simulink model "Basics"  (R2019a)
settings: Solver=ode1  StartTime=0.0  StopTime=2.5  FixedStep=Ts_Power  RelTol=1e-3
PostLoadFcn:
  | %% Init for wind PnO models - global system parameters
  | OVERRIDE_SSN_MEMORY_LIMIT=1;
  | Ts=50e-6;
  | % Ts=50e-10;
  | Ts_Power=Ts;
  | Ts_Control=2*Ts;
  | freq = 50;
  | Fnom=freq;
  | Vac=400e3;
InitFcn:
  | %% Init for wind PnO models - global system parameters
  | OVERRIDE_SSN_MEMORY_LIMIT=1;
  | Ts=50e-6;
  | % Ts=50e-10;
  | Ts_Power=Ts;
  | Ts_Control=2*Ts;
  | freq = 50;
  | Fnom=freq;
  | Vac=225e3;
values from neighbouring files (symbols this model uses):
  ohl_posCap = 11.33e-009/2    (= 5.665e-09)    [variable.m]
  ohl_posInd = 1.05e-3/2    (= 0.000525)    [variable.m]
  ohl_posR = 0.1153/2    (= 0.05765)    [variable.m]
  ohl_zeroCap = 5.01e-009/2    (= 2.505e-09)    [variable.m]
  ohl_zeroInd = 3.32e-3/2    (= 0.00166)    [variable.m]
  ohl_zeroR = 0.4138/2    (= 0.2069)    [variable.m]
  sub_posCap = 0.16e-006    (= 1.6e-07)    [variable.m]
  sub_posInd = 0.001400563    [variable.m]
  sub_posR = 0.036    [variable.m]
  sub_zeroCap = 0.053333e-006    (= 5.3333e-08)    [variable.m]
  sub_zeroInd = 0.00420169    [variable.m]
  sub_zeroR = 0.108    [variable.m]
  transfo_L1 = 0.05999374    [variable.m]
  transfo_L2 = 0.05999374    [variable.m]
  transfo_R1 = 0.000866667    [variable.m]
  transfo_R2 = 0.00086667    [variable.m]
undefined symbols (not defined in the file or in its folder): D1, D11, Delta, den, DiscIntNeverNeededParam, dx, find_system, gcbh, num, out_Buses, out_WindFarms, sps_rtmsupport
libraries: powerlib x173, simulink x80, powerlib_meascontrol x80, elements x52, eeSinusoidalMeasurement x46, simulink_extras x40, spsVIMeasurementModel x36, eePowerMeasurement x15
(part 21 of 22)

== system Basics/SM_WT1/Wind Type IV Detailed v2.1 - 3/Control/Measurement and Transformation/Discrete 3-phase PLL-Driven Positive-Sequence Active & Reactive Power/Discrete 3-phase PLL-Driven Positive-Sequence Fundamental Value/Discrete Variable Frequency Mean value1 ==
  note: Pierre Giroux, Gilbert Sybille, Richard Gagnon
      | Power System Simulation Laboratory
      | IREQ, Hydro-Quebc
  note: Variable frequency - Discrete Mean Value
  Freq : Inport  PortDimensions=1
  In : Inport  Port=2  PortDimensions=1
  Correction subsystem : Subsystem
  Discrete Variable Transport Delay : Subsystem  mask(Discrete variable transport delay){MaxDelay=MaxDelay, InitialValue=0, Ts=Ts}
      mask prompts: MaxDelay "Maximum delay (s):"; InitialValue "Initial input:"; Ts "Sample time:"
      mask help:
      | Apply a delay to the first input (In) signal.
      | The second input (D) specifies the delay time.
  Gain : Gain  Gain=Ts  SaturateOnIntegerOverflow=on  OutDataTypeStr=Inherit: Same as input  ParamDataTypeStr=Inherit: Same as input
  Integ4 : DiscreteIntegrator  IntegratorMethod=Integration: Trapezoidal  SampleTime=Ts  ICPrevOutput=DiscIntNeverNeededParam  ICPrevScaledInput=DiscIntNeverNeededParam
  Number of samples per cycle : Fcn  Expr=1/u[1]/Ts
  Product : Product  SaturateOnIntegerOverflow=on  InputSameDT=on  OutDataTypeStr=Inherit: Same as first input
  Rounding Function : Rounding  Operator=ceil
  Step : Step  Time=1/Finit  SampleTime=Ts
  Sum5 : Sum  SaturateOnIntegerOverflow=on  InputSameDT=on  OutDataTypeStr=Inherit: Same as first input
  Sum7 : Sum  Inputs=-+  SaturateOnIntegerOverflow=on  InputSameDT=on  OutDataTypeStr=Inherit: Same as first input
  Switch : Switch  Threshold=0.5  InputSameDT=on
  To avoid division by zero : Saturate  UpperLimit=1e6  LowerLimit=1e-6
  Unit Delay : UnitDelay  InitialCondition=Vinit  SampleTime=Ts  HasFrameUpgradeWarning=on
  Mean : Outport  VectorParamsAs1DForOutWhenUnconnected=on
  wires:
  In/1 -> Integ4/1, Correction subsystem/3(In)  "In"
  Product/1 -> Sum5/1  "Mean value"
  Discrete Variable Transport Delay/1(Out) -> Sum7/1
  Sum7/1 -> Product/1
  Integ4/1 -> Discrete Variable Transport Delay/1(In), Sum7/2
  Freq/1 -> Product/2, To avoid division by zero/1  "Freq"
  Gain/1 -> Discrete Variable Transport Delay/2(D)  "Delay"
  Rounding Function/1 -> Gain/1, Correction subsystem/2(F)
  Number of samples per cycle/1 -> Rounding Function/1, Correction subsystem/1(N)
  Sum5/1 -> Switch/1
  Unit Delay/1 -> Switch/3
  Switch/1 -> Mean/1, Unit Delay/1
  To avoid division by zero/1 -> Number of samples per cycle/1  "Freq"
  Correction subsystem/1(Out) -> Sum5/2
  Step/1 -> Switch/2

== system Basics/SM_WT1/Wind Type IV Detailed v2.1 - 3/Control/Measurement and Transformation/Discrete 3-phase PLL-Driven Positive-Sequence Active & Reactive Power/Discrete 3-phase PLL-Driven Positive-Sequence Fundamental Value/Discrete Variable Frequency Mean value2 ==
  note: Variable frequency - Discrete Mean Value
  note: Pierre Giroux, Gilbert Sybille, Richard Gagnon
      | Power System Simulation Laboratory
      | IREQ, Hydro-Quebc
  Freq : Inport  PortDimensions=1
  In : Inport  Port=2  PortDimensions=1
  Correction subsystem : Subsystem
  Discrete Variable Transport Delay : Subsystem  mask(Discrete variable transport delay){MaxDelay=MaxDelay, InitialValue=0, Ts=Ts}
      mask prompts: MaxDelay "Maximum delay (s):"; InitialValue "Initial input:"; Ts "Sample time:"
      mask help:
      | Apply a delay to the first input (In) signal.
      | The second input (D) specifies the delay time.
  Gain : Gain  Gain=Ts  SaturateOnIntegerOverflow=on  OutDataTypeStr=Inherit: Same as input  ParamDataTypeStr=Inherit: Same as input
  Integ4 : DiscreteIntegrator  IntegratorMethod=Integration: Trapezoidal  SampleTime=Ts  ICPrevOutput=DiscIntNeverNeededParam  ICPrevScaledInput=DiscIntNeverNeededParam
  Number of samples per cycle : Fcn  Expr=1/u[1]/Ts
  Product : Product  SaturateOnIntegerOverflow=on  InputSameDT=on  OutDataTypeStr=Inherit: Same as first input
  Rounding Function : Rounding  Operator=ceil
  Step : Step  Time=1/Finit  SampleTime=Ts
  Sum5 : Sum  SaturateOnIntegerOverflow=on  InputSameDT=on  OutDataTypeStr=Inherit: Same as first input
  Sum7 : Sum  Inputs=-+  SaturateOnIntegerOverflow=on  InputSameDT=on  OutDataTypeStr=Inherit: Same as first input
  Switch : Switch  Threshold=0.5  InputSameDT=on
  To avoid division by zero : Saturate  UpperLimit=1e6  LowerLimit=1e-6
  Unit Delay : UnitDelay  InitialCondition=Vinit  SampleTime=Ts  HasFrameUpgradeWarning=on
  Mean : Outport  VectorParamsAs1DForOutWhenUnconnected=on
  wires:
  Step/1 -> Switch/2
  Correction subsystem/1(Out) -> Sum5/2
  To avoid division by zero/1 -> Number of samples per cycle/1  "Freq"
  Switch/1 -> Unit Delay/1, Mean/1
  Unit Delay/1 -> Switch/3
  Sum5/1 -> Switch/1
  Number of samples per cycle/1 -> Correction subsystem/1(N), Rounding Function/1
  Rounding Function/1 -> Correction subsystem/2(F), Gain/1
  Gain/1 -> Discrete Variable Transport Delay/2(D)  "Delay"
  Freq/1 -> To avoid division by zero/1, Product/2  "Freq"
  Integ4/1 -> Sum7/2, Discrete Variable Transport Delay/1(In)
  Sum7/1 -> Product/1
  Discrete Variable Transport Delay/1(Out) -> Sum7/1
  Product/1 -> Sum5/1  "Mean value"
  In/1 -> Correction subsystem/3(In), Integ4/1  "In"

== system Basics/SM_WT1/Wind Type IV Detailed v2.1 - 3/Control/Measurement and Transformation/Discrete 3-phase PLL-Driven Positive-Sequence Active & Reactive Power/Discrete 3-phase PLL-Driven Positive-Sequence Fundamental Value2/Discrete Variable Frequency Mean value1 ==
  note: Variable frequency - Discrete Mean Value
  note: Pierre Giroux, Gilbert Sybille, Richard Gagnon
      | Power System Simulation Laboratory
      | IREQ, Hydro-Quebc
  Freq : Inport  PortDimensions=1
  In : Inport  Port=2  PortDimensions=1
  Correction subsystem : Subsystem
  Discrete Variable Transport Delay : Subsystem  mask(Discrete variable transport delay){MaxDelay=MaxDelay, InitialValue=0, Ts=Ts}
      mask prompts: MaxDelay "Maximum delay (s):"; InitialValue "Initial input:"; Ts "Sample time:"
      mask help:
      | Apply a delay to the first input (In) signal.
      | The second input (D) specifies the delay time.
  Gain : Gain  Gain=Ts  SaturateOnIntegerOverflow=on  OutDataTypeStr=Inherit: Same as input  ParamDataTypeStr=Inherit: Same as input
  Integ4 : DiscreteIntegrator  IntegratorMethod=Integration: Trapezoidal  SampleTime=Ts  ICPrevOutput=DiscIntNeverNeededParam  ICPrevScaledInput=DiscIntNeverNeededParam
  Number of samples per cycle : Fcn  Expr=1/u[1]/Ts
  Product : Product  SaturateOnIntegerOverflow=on  InputSameDT=on  OutDataTypeStr=Inherit: Same as first input
  Rounding Function : Rounding  Operator=ceil
  Step : Step  Time=1/Finit  SampleTime=Ts
  Sum5 : Sum  SaturateOnIntegerOverflow=on  InputSameDT=on  OutDataTypeStr=Inherit: Same as first input
  Sum7 : Sum  Inputs=-+  SaturateOnIntegerOverflow=on  InputSameDT=on  OutDataTypeStr=Inherit: Same as first input
  Switch : Switch  Threshold=0.5  InputSameDT=on
  To avoid division by zero : Saturate  UpperLimit=1e6  LowerLimit=1e-6
  Unit Delay : UnitDelay  InitialCondition=Vinit  SampleTime=Ts  HasFrameUpgradeWarning=on
  Mean : Outport  VectorParamsAs1DForOutWhenUnconnected=on
  wires:
  Step/1 -> Switch/2
  Correction subsystem/1(Out) -> Sum5/2
  To avoid division by zero/1 -> Number of samples per cycle/1  "Freq"
  Switch/1 -> Unit Delay/1, Mean/1
  Unit Delay/1 -> Switch/3
  Sum5/1 -> Switch/1
  Number of samples per cycle/1 -> Correction subsystem/1(N), Rounding Function/1
  Rounding Function/1 -> Correction subsystem/2(F), Gain/1
  Gain/1 -> Discrete Variable Transport Delay/2(D)  "Delay"
  Freq/1 -> To avoid division by zero/1, Product/2  "Freq"
  Integ4/1 -> Sum7/2, Discrete Variable Transport Delay/1(In)
  Sum7/1 -> Product/1
  Discrete Variable Transport Delay/1(Out) -> Sum7/1
  Product/1 -> Sum5/1  "Mean value"
  In/1 -> Correction subsystem/3(In), Integ4/1  "In"

== system Basics/SM_WT1/Wind Type IV Detailed v2.1 - 3/Control/Measurement and Transformation/Discrete 3-phase PLL-Driven Positive-Sequence Active & Reactive Power/Discrete 3-phase PLL-Driven Positive-Sequence Fundamental Value2/Discrete Variable Frequency Mean value2 ==
  note: Pierre Giroux, Gilbert Sybille, Richard Gagnon
      | Power System Simulation Laboratory
      | IREQ, Hydro-Quebc
  note: Variable frequency - Discrete Mean Value
  Freq : Inport  PortDimensions=1
  In : Inport  Port=2  PortDimensions=1
  Correction subsystem : Subsystem
  Discrete Variable Transport Delay : Subsystem  mask(Discrete variable transport delay){MaxDelay=MaxDelay, InitialValue=0, Ts=Ts}
      mask prompts: MaxDelay "Maximum delay (s):"; InitialValue "Initial input:"; Ts "Sample time:"
      mask help:
      | Apply a delay to the first input (In) signal.
      | The second input (D) specifies the delay time.
  Gain : Gain  Gain=Ts  SaturateOnIntegerOverflow=on  OutDataTypeStr=Inherit: Same as input  ParamDataTypeStr=Inherit: Same as input
  Integ4 : DiscreteIntegrator  IntegratorMethod=Integration: Trapezoidal  SampleTime=Ts  ICPrevOutput=DiscIntNeverNeededParam  ICPrevScaledInput=DiscIntNeverNeededParam
  Number of samples per cycle : Fcn  Expr=1/u[1]/Ts
  Product : Product  SaturateOnIntegerOverflow=on  InputSameDT=on  OutDataTypeStr=Inherit: Same as first input
  Rounding Function : Rounding  Operator=ceil
  Step : Step  Time=1/Finit  SampleTime=Ts
  Sum5 : Sum  SaturateOnIntegerOverflow=on  InputSameDT=on  OutDataTypeStr=Inherit: Same as first input
  Sum7 : Sum  Inputs=-+  SaturateOnIntegerOverflow=on  InputSameDT=on  OutDataTypeStr=Inherit: Same as first input
  Switch : Switch  Threshold=0.5  InputSameDT=on
  To avoid division by zero : Saturate  UpperLimit=1e6  LowerLimit=1e-6
  Unit Delay : UnitDelay  InitialCondition=Vinit  SampleTime=Ts  HasFrameUpgradeWarning=on
  Mean : Outport  VectorParamsAs1DForOutWhenUnconnected=on
  wires:
  In/1 -> Integ4/1, Correction subsystem/3(In)  "In"
  Product/1 -> Sum5/1  "Mean value"
  Discrete Variable Transport Delay/1(Out) -> Sum7/1
  Sum7/1 -> Product/1
  Integ4/1 -> Discrete Variable Transport Delay/1(In), Sum7/2
  Freq/1 -> Product/2, To avoid division by zero/1  "Freq"
  Gain/1 -> Discrete Variable Transport Delay/2(D)  "Delay"
  Rounding Function/1 -> Gain/1, Correction subsystem/2(F)
  Number of samples per cycle/1 -> Rounding Function/1, Correction subsystem/1(N)
  Sum5/1 -> Switch/1
  Unit Delay/1 -> Switch/3
  Switch/1 -> Mean/1, Unit Delay/1
  To avoid division by zero/1 -> Number of samples per cycle/1  "Freq"
  Correction subsystem/1(Out) -> Sum5/2
  Step/1 -> Switch/2

== system Basics/SM_WT1/Wind Type IV Detailed v2.1 - 7/Control/Measurement and Transformation/Discrete 3-phase PLL-Driven Positive-Sequence Active & Reactive Power/Discrete 3-phase PLL-Driven Positive-Sequence Fundamental Value/Discrete Variable Frequency Mean value1 ==
  note: Variable frequency - Discrete Mean Value
  note: Pierre Giroux, Gilbert Sybille, Richard Gagnon
      | Power System Simulation Laboratory
      | IREQ, Hydro-Quebc
  Freq : Inport  PortDimensions=1
  In : Inport  Port=2  PortDimensions=1
  Correction subsystem : Subsystem
  Discrete Variable Transport Delay : Subsystem  mask(Discrete variable transport delay){MaxDelay=MaxDelay, InitialValue=0, Ts=Ts}
      mask prompts: MaxDelay "Maximum delay (s):"; InitialValue "Initial input:"; Ts "Sample time:"
      mask help:
      | Apply a delay to the first input (In) signal.
      | The second input (D) specifies the delay time.
  Gain : Gain  Gain=Ts  SaturateOnIntegerOverflow=on  OutDataTypeStr=Inherit: Same as input  ParamDataTypeStr=Inherit: Same as input
  Integ4 : DiscreteIntegrator  IntegratorMethod=Integration: Trapezoidal  SampleTime=Ts  ICPrevOutput=DiscIntNeverNeededParam  ICPrevScaledInput=DiscIntNeverNeededParam
  Number of samples per cycle : Fcn  Expr=1/u[1]/Ts
  Product : Product  SaturateOnIntegerOverflow=on  InputSameDT=on  OutDataTypeStr=Inherit: Same as first input
  Rounding Function : Rounding  Operator=ceil
  Step : Step  Time=1/Finit  SampleTime=Ts
  Sum5 : Sum  SaturateOnIntegerOverflow=on  InputSameDT=on  OutDataTypeStr=Inherit: Same as first input
  Sum7 : Sum  Inputs=-+  SaturateOnIntegerOverflow=on  InputSameDT=on  OutDataTypeStr=Inherit: Same as first input
  Switch : Switch  Threshold=0.5  InputSameDT=on
  To avoid division by zero : Saturate  UpperLimit=1e6  LowerLimit=1e-6
  Unit Delay : UnitDelay  InitialCondition=Vinit  SampleTime=Ts  HasFrameUpgradeWarning=on
  Mean : Outport  VectorParamsAs1DForOutWhenUnconnected=on
  wires:
  Step/1 -> Switch/2
  Correction subsystem/1(Out) -> Sum5/2
  To avoid division by zero/1 -> Number of samples per cycle/1  "Freq"
  Switch/1 -> Unit Delay/1, Mean/1
  Unit Delay/1 -> Switch/3
  Sum5/1 -> Switch/1
  Number of samples per cycle/1 -> Correction subsystem/1(N), Rounding Function/1
  Rounding Function/1 -> Correction subsystem/2(F), Gain/1
  Gain/1 -> Discrete Variable Transport Delay/2(D)  "Delay"
  Freq/1 -> To avoid division by zero/1, Product/2  "Freq"
  Integ4/1 -> Sum7/2, Discrete Variable Transport Delay/1(In)
  Sum7/1 -> Product/1
  Discrete Variable Transport Delay/1(Out) -> Sum7/1
  Product/1 -> Sum5/1  "Mean value"
  In/1 -> Correction subsystem/3(In), Integ4/1  "In"

== system Basics/SM_WT1/Wind Type IV Detailed v2.1 - 7/Control/Measurement and Transformation/Discrete 3-phase PLL-Driven Positive-Sequence Active & Reactive Power/Discrete 3-phase PLL-Driven Positive-Sequence Fundamental Value/Discrete Variable Frequency Mean value2 ==
  note: Pierre Giroux, Gilbert Sybille, Richard Gagnon
      | Power System Simulation Laboratory
      | IREQ, Hydro-Quebc
  note: Variable frequency - Discrete Mean Value
  Freq : Inport  PortDimensions=1
  In : Inport  Port=2  PortDimensions=1
  Correction subsystem : Subsystem
  Discrete Variable Transport Delay : Subsystem  mask(Discrete variable transport delay){MaxDelay=MaxDelay, InitialValue=0, Ts=Ts}
      mask prompts: MaxDelay "Maximum delay (s):"; InitialValue "Initial input:"; Ts "Sample time:"
      mask help:
      | Apply a delay to the first input (In) signal.
      | The second input (D) specifies the delay time.
  Gain : Gain  Gain=Ts  SaturateOnIntegerOverflow=on  OutDataTypeStr=Inherit: Same as input  ParamDataTypeStr=Inherit: Same as input
  Integ4 : DiscreteIntegrator  IntegratorMethod=Integration: Trapezoidal  SampleTime=Ts  ICPrevOutput=DiscIntNeverNeededParam  ICPrevScaledInput=DiscIntNeverNeededParam
  Number of samples per cycle : Fcn  Expr=1/u[1]/Ts
  Product : Product  SaturateOnIntegerOverflow=on  InputSameDT=on  OutDataTypeStr=Inherit: Same as first input
  Rounding Function : Rounding  Operator=ceil
  Step : Step  Time=1/Finit  SampleTime=Ts
  Sum5 : Sum  SaturateOnIntegerOverflow=on  InputSameDT=on  OutDataTypeStr=Inherit: Same as first input
  Sum7 : Sum  Inputs=-+  SaturateOnIntegerOverflow=on  InputSameDT=on  OutDataTypeStr=Inherit: Same as first input
  Switch : Switch  Threshold=0.5  InputSameDT=on
  To avoid division by zero : Saturate  UpperLimit=1e6  LowerLimit=1e-6
  Unit Delay : UnitDelay  InitialCondition=Vinit  SampleTime=Ts  HasFrameUpgradeWarning=on
  Mean : Outport  VectorParamsAs1DForOutWhenUnconnected=on
  wires:
  In/1 -> Integ4/1, Correction subsystem/3(In)  "In"
  Product/1 -> Sum5/1  "Mean value"
  Discrete Variable Transport Delay/1(Out) -> Sum7/1
  Sum7/1 -> Product/1
  Integ4/1 -> Discrete Variable Transport Delay/1(In), Sum7/2
  Freq/1 -> Product/2, To avoid division by zero/1  "Freq"
  Gain/1 -> Discrete Variable Transport Delay/2(D)  "Delay"
  Rounding Function/1 -> Gain/1, Correction subsystem/2(F)
  Number of samples per cycle/1 -> Rounding Function/1, Correction subsystem/1(N)
  Sum5/1 -> Switch/1
  Unit Delay/1 -> Switch/3
  Switch/1 -> Mean/1, Unit Delay/1
  To avoid division by zero/1 -> Number of samples per cycle/1  "Freq"
  Correction subsystem/1(Out) -> Sum5/2
  Step/1 -> Switch/2

== system Basics/SM_WT1/Wind Type IV Detailed v2.1 - 7/Control/Measurement and Transformation/Discrete 3-phase PLL-Driven Positive-Sequence Active & Reactive Power/Discrete 3-phase PLL-Driven Positive-Sequence Fundamental Value2/Discrete Variable Frequency Mean value1 ==
  note: Pierre Giroux, Gilbert Sybille, Richard Gagnon
      | Power System Simulation Laboratory
      | IREQ, Hydro-Quebc
  note: Variable frequency - Discrete Mean Value
  Freq : Inport  PortDimensions=1
  In : Inport  Port=2  PortDimensions=1
  Correction subsystem : Subsystem
  Discrete Variable Transport Delay : Subsystem  mask(Discrete variable transport delay){MaxDelay=MaxDelay, InitialValue=0, Ts=Ts}
      mask prompts: MaxDelay "Maximum delay (s):"; InitialValue "Initial input:"; Ts "Sample time:"
      mask help:
      | Apply a delay to the first input (In) signal.
      | The second input (D) specifies the delay time.
  Gain : Gain  Gain=Ts  SaturateOnIntegerOverflow=on  OutDataTypeStr=Inherit: Same as input  ParamDataTypeStr=Inherit: Same as input
  Integ4 : DiscreteIntegrator  IntegratorMethod=Integration: Trapezoidal  SampleTime=Ts  ICPrevOutput=DiscIntNeverNeededParam  ICPrevScaledInput=DiscIntNeverNeededParam
  Number of samples per cycle : Fcn  Expr=1/u[1]/Ts
  Product : Product  SaturateOnIntegerOverflow=on  InputSameDT=on  OutDataTypeStr=Inherit: Same as first input
  Rounding Function : Rounding  Operator=ceil
  Step : Step  Time=1/Finit  SampleTime=Ts
  Sum5 : Sum  SaturateOnIntegerOverflow=on  InputSameDT=on  OutDataTypeStr=Inherit: Same as first input
  Sum7 : Sum  Inputs=-+  SaturateOnIntegerOverflow=on  InputSameDT=on  OutDataTypeStr=Inherit: Same as first input
  Switch : Switch  Threshold=0.5  InputSameDT=on
  To avoid division by zero : Saturate  UpperLimit=1e6  LowerLimit=1e-6
  Unit Delay : UnitDelay  InitialCondition=Vinit  SampleTime=Ts  HasFrameUpgradeWarning=on
  Mean : Outport  VectorParamsAs1DForOutWhenUnconnected=on
  wires:
  In/1 -> Integ4/1, Correction subsystem/3(In)  "In"
  Product/1 -> Sum5/1  "Mean value"
  Discrete Variable Transport Delay/1(Out) -> Sum7/1
  Sum7/1 -> Product/1
  Integ4/1 -> Discrete Variable Transport Delay/1(In), Sum7/2
  Freq/1 -> Product/2, To avoid division by zero/1  "Freq"
  Gain/1 -> Discrete Variable Transport Delay/2(D)  "Delay"
  Rounding Function/1 -> Gain/1, Correction subsystem/2(F)
  Number of samples per cycle/1 -> Rounding Function/1, Correction subsystem/1(N)
  Sum5/1 -> Switch/1
  Unit Delay/1 -> Switch/3
  Switch/1 -> Mean/1, Unit Delay/1
  To avoid division by zero/1 -> Number of samples per cycle/1  "Freq"
  Correction subsystem/1(Out) -> Sum5/2
  Step/1 -> Switch/2

== system Basics/SM_WT1/Wind Type IV Detailed v2.1 - 7/Control/Measurement and Transformation/Discrete 3-phase PLL-Driven Positive-Sequence Active & Reactive Power/Discrete 3-phase PLL-Driven Positive-Sequence Fundamental Value2/Discrete Variable Frequency Mean value2 ==
  note: Variable frequency - Discrete Mean Value
  note: Pierre Giroux, Gilbert Sybille, Richard Gagnon
      | Power System Simulation Laboratory
      | IREQ, Hydro-Quebc
  Freq : Inport  PortDimensions=1
  In : Inport  Port=2  PortDimensions=1
  Correction subsystem : Subsystem
  Discrete Variable Transport Delay : Subsystem  mask(Discrete variable transport delay){MaxDelay=MaxDelay, InitialValue=0, Ts=Ts}
      mask prompts: MaxDelay "Maximum delay (s):"; InitialValue "Initial input:"; Ts "Sample time:"
      mask help:
      | Apply a delay to the first input (In) signal.
      | The second input (D) specifies the delay time.
  Gain : Gain  Gain=Ts  SaturateOnIntegerOverflow=on  OutDataTypeStr=Inherit: Same as input  ParamDataTypeStr=Inherit: Same as input
  Integ4 : DiscreteIntegrator  IntegratorMethod=Integration: Trapezoidal  SampleTime=Ts  ICPrevOutput=DiscIntNeverNeededParam  ICPrevScaledInput=DiscIntNeverNeededParam
  Number of samples per cycle : Fcn  Expr=1/u[1]/Ts
  Product : Product  SaturateOnIntegerOverflow=on  InputSameDT=on  OutDataTypeStr=Inherit: Same as first input
  Rounding Function : Rounding  Operator=ceil
  Step : Step  Time=1/Finit  SampleTime=Ts
  Sum5 : Sum  SaturateOnIntegerOverflow=on  InputSameDT=on  OutDataTypeStr=Inherit: Same as first input
  Sum7 : Sum  Inputs=-+  SaturateOnIntegerOverflow=on  InputSameDT=on  OutDataTypeStr=Inherit: Same as first input
  Switch : Switch  Threshold=0.5  InputSameDT=on
  To avoid division by zero : Saturate  UpperLimit=1e6  LowerLimit=1e-6
  Unit Delay : UnitDelay  InitialCondition=Vinit  SampleTime=Ts  HasFrameUpgradeWarning=on
  Mean : Outport  VectorParamsAs1DForOutWhenUnconnected=on
  wires:
  Step/1 -> Switch/2
  Correction subsystem/1(Out) -> Sum5/2
  To avoid division by zero/1 -> Number of samples per cycle/1  "Freq"
  Switch/1 -> Unit Delay/1, Mean/1
  Unit Delay/1 -> Switch/3
  Sum5/1 -> Switch/1
  Number of samples per cycle/1 -> Correction subsystem/1(N), Rounding Function/1
  Rounding Function/1 -> Correction subsystem/2(F), Gain/1
  Gain/1 -> Discrete Variable Transport Delay/2(D)  "Delay"
  Freq/1 -> To avoid division by zero/1, Product/2  "Freq"
  Integ4/1 -> Sum7/2, Discrete Variable Transport Delay/1(In)
  Sum7/1 -> Product/1
  Discrete Variable Transport Delay/1(Out) -> Sum7/1
  Product/1 -> Sum5/1  "Mean value"
  In/1 -> Correction subsystem/3(In), Integ4/1  "In"

== system Basics/SM_WT1/Wind Type IV Detailed v2.1 - 9/Control/Measurement and Transformation/Discrete 3-phase PLL-Driven Positive-Sequence Active & Reactive Power/Discrete 3-phase PLL-Driven Positive-Sequence Fundamental Value/Discrete Variable Frequency Mean value1 ==
  note: Variable frequency - Discrete Mean Value
  note: Pierre Giroux, Gilbert Sybille, Richard Gagnon
      | Power System Simulation Laboratory
      | IREQ, Hydro-Quebc
  Freq : Inport  PortDimensions=1
  In : Inport  Port=2  PortDimensions=1
  Correction subsystem : Subsystem
  Discrete Variable Transport Delay : Subsystem  mask(Discrete variable transport delay){MaxDelay=MaxDelay, InitialValue=0, Ts=Ts}
      mask prompts: MaxDelay "Maximum delay (s):"; InitialValue "Initial input:"; Ts "Sample time:"
      mask help:
      | Apply a delay to the first input (In) signal.
      | The second input (D) specifies the delay time.
  Gain : Gain  Gain=Ts  SaturateOnIntegerOverflow=on  OutDataTypeStr=Inherit: Same as input  ParamDataTypeStr=Inherit: Same as input
  Integ4 : DiscreteIntegrator  IntegratorMethod=Integration: Trapezoidal  SampleTime=Ts  ICPrevOutput=DiscIntNeverNeededParam  ICPrevScaledInput=DiscIntNeverNeededParam
  Number of samples per cycle : Fcn  Expr=1/u[1]/Ts
  Product : Product  SaturateOnIntegerOverflow=on  InputSameDT=on  OutDataTypeStr=Inherit: Same as first input
  Rounding Function : Rounding  Operator=ceil
  Step : Step  Time=1/Finit  SampleTime=Ts
  Sum5 : Sum  SaturateOnIntegerOverflow=on  InputSameDT=on  OutDataTypeStr=Inherit: Same as first input
  Sum7 : Sum  Inputs=-+  SaturateOnIntegerOverflow=on  InputSameDT=on  OutDataTypeStr=Inherit: Same as first input
  Switch : Switch  Threshold=0.5  InputSameDT=on
  To avoid division by zero : Saturate  UpperLimit=1e6  LowerLimit=1e-6
  Unit Delay : UnitDelay  InitialCondition=Vinit  SampleTime=Ts  HasFrameUpgradeWarning=on
  Mean : Outport  VectorParamsAs1DForOutWhenUnconnected=on
  wires:
  Step/1 -> Switch/2
  Correction subsystem/1(Out) -> Sum5/2
  To avoid division by zero/1 -> Number of samples per cycle/1  "Freq"
  Switch/1 -> Unit Delay/1, Mean/1
  Unit Delay/1 -> Switch/3
  Sum5/1 -> Switch/1
  Number of samples per cycle/1 -> Correction subsystem/1(N), Rounding Function/1
  Rounding Function/1 -> Correction subsystem/2(F), Gain/1
  Gain/1 -> Discrete Variable Transport Delay/2(D)  "Delay"
  Freq/1 -> To avoid division by zero/1, Product/2  "Freq"
  Integ4/1 -> Sum7/2, Discrete Variable Transport Delay/1(In)
  Sum7/1 -> Product/1
  Discrete Variable Transport Delay/1(Out) -> Sum7/1
  Product/1 -> Sum5/1  "Mean value"
  In/1 -> Correction subsystem/3(In), Integ4/1  "In"

== system Basics/SM_WT1/Wind Type IV Detailed v2.1 - 9/Control/Measurement and Transformation/Discrete 3-phase PLL-Driven Positive-Sequence Active & Reactive Power/Discrete 3-phase PLL-Driven Positive-Sequence Fundamental Value/Discrete Variable Frequency Mean value2 ==
  note: Pierre Giroux, Gilbert Sybille, Richard Gagnon
      | Power System Simulation Laboratory
      | IREQ, Hydro-Quebc
  note: Variable frequency - Discrete Mean Value
  Freq : Inport  PortDimensions=1
  In : Inport  Port=2  PortDimensions=1
  Correction subsystem : Subsystem
  Discrete Variable Transport Delay : Subsystem  mask(Discrete variable transport delay){MaxDelay=MaxDelay, InitialValue=0, Ts=Ts}
      mask prompts: MaxDelay "Maximum delay (s):"; InitialValue "Initial input:"; Ts "Sample time:"
      mask help:
      | Apply a delay to the first input (In) signal.
      | The second input (D) specifies the delay time.
  Gain : Gain  Gain=Ts  SaturateOnIntegerOverflow=on  OutDataTypeStr=Inherit: Same as input  ParamDataTypeStr=Inherit: Same as input
  Integ4 : DiscreteIntegrator  IntegratorMethod=Integration: Trapezoidal  SampleTime=Ts  ICPrevOutput=DiscIntNeverNeededParam  ICPrevScaledInput=DiscIntNeverNeededParam
  Number of samples per cycle : Fcn  Expr=1/u[1]/Ts
  Product : Product  SaturateOnIntegerOverflow=on  InputSameDT=on  OutDataTypeStr=Inherit: Same as first input
  Rounding Function : Rounding  Operator=ceil
  Step : Step  Time=1/Finit  SampleTime=Ts
  Sum5 : Sum  SaturateOnIntegerOverflow=on  InputSameDT=on  OutDataTypeStr=Inherit: Same as first input
  Sum7 : Sum  Inputs=-+  SaturateOnIntegerOverflow=on  InputSameDT=on  OutDataTypeStr=Inherit: Same as first input
  Switch : Switch  Threshold=0.5  InputSameDT=on
  To avoid division by zero : Saturate  UpperLimit=1e6  LowerLimit=1e-6
  Unit Delay : UnitDelay  InitialCondition=Vinit  SampleTime=Ts  HasFrameUpgradeWarning=on
  Mean : Outport  VectorParamsAs1DForOutWhenUnconnected=on
  wires:
  In/1 -> Integ4/1, Correction subsystem/3(In)  "In"
  Product/1 -> Sum5/1  "Mean value"
  Discrete Variable Transport Delay/1(Out) -> Sum7/1
  Sum7/1 -> Product/1
  Integ4/1 -> Discrete Variable Transport Delay/1(In), Sum7/2
  Freq/1 -> Product/2, To avoid division by zero/1  "Freq"
  Gain/1 -> Discrete Variable Transport Delay/2(D)  "Delay"
  Rounding Function/1 -> Gain/1, Correction subsystem/2(F)
  Number of samples per cycle/1 -> Rounding Function/1, Correction subsystem/1(N)
  Sum5/1 -> Switch/1
  Unit Delay/1 -> Switch/3
  Switch/1 -> Mean/1, Unit Delay/1
  To avoid division by zero/1 -> Number of samples per cycle/1  "Freq"
  Correction subsystem/1(Out) -> Sum5/2
  Step/1 -> Switch/2

== system Basics/SM_WT1/Wind Type IV Detailed v2.1 - 9/Control/Measurement and Transformation/Discrete 3-phase PLL-Driven Positive-Sequence Active & Reactive Power/Discrete 3-phase PLL-Driven Positive-Sequence Fundamental Value2/Discrete Variable Frequency Mean value1 ==
  note: Pierre Giroux, Gilbert Sybille, Richard Gagnon
      | Power System Simulation Laboratory
      | IREQ, Hydro-Quebc
  note: Variable frequency - Discrete Mean Value
  Freq : Inport  PortDimensions=1
  In : Inport  Port=2  PortDimensions=1
  Correction subsystem : Subsystem
  Discrete Variable Transport Delay : Subsystem  mask(Discrete variable transport delay){MaxDelay=MaxDelay, InitialValue=0, Ts=Ts}
      mask prompts: MaxDelay "Maximum delay (s):"; InitialValue "Initial input:"; Ts "Sample time:"
      mask help:
      | Apply a delay to the first input (In) signal.
      | The second input (D) specifies the delay time.
  Gain : Gain  Gain=Ts  SaturateOnIntegerOverflow=on  OutDataTypeStr=Inherit: Same as input  ParamDataTypeStr=Inherit: Same as input
  Integ4 : DiscreteIntegrator  IntegratorMethod=Integration: Trapezoidal  SampleTime=Ts  ICPrevOutput=DiscIntNeverNeededParam  ICPrevScaledInput=DiscIntNeverNeededParam
  Number of samples per cycle : Fcn  Expr=1/u[1]/Ts
  Product : Product  SaturateOnIntegerOverflow=on  InputSameDT=on  OutDataTypeStr=Inherit: Same as first input
  Rounding Function : Rounding  Operator=ceil
  Step : Step  Time=1/Finit  SampleTime=Ts
  Sum5 : Sum  SaturateOnIntegerOverflow=on  InputSameDT=on  OutDataTypeStr=Inherit: Same as first input
  Sum7 : Sum  Inputs=-+  SaturateOnIntegerOverflow=on  InputSameDT=on  OutDataTypeStr=Inherit: Same as first input
  Switch : Switch  Threshold=0.5  InputSameDT=on
  To avoid division by zero : Saturate  UpperLimit=1e6  LowerLimit=1e-6
  Unit Delay : UnitDelay  InitialCondition=Vinit  SampleTime=Ts  HasFrameUpgradeWarning=on
  Mean : Outport  VectorParamsAs1DForOutWhenUnconnected=on
  wires:
  In/1 -> Integ4/1, Correction subsystem/3(In)  "In"
  Product/1 -> Sum5/1  "Mean value"
  Discrete Variable Transport Delay/1(Out) -> Sum7/1
  Sum7/1 -> Product/1
  Integ4/1 -> Discrete Variable Transport Delay/1(In), Sum7/2
  Freq/1 -> Product/2, To avoid division by zero/1  "Freq"
  Gain/1 -> Discrete Variable Transport Delay/2(D)  "Delay"
  Rounding Function/1 -> Gain/1, Correction subsystem/2(F)
  Number of samples per cycle/1 -> Rounding Function/1, Correction subsystem/1(N)
  Sum5/1 -> Switch/1
  Unit Delay/1 -> Switch/3
  Switch/1 -> Mean/1, Unit Delay/1
  To avoid division by zero/1 -> Number of samples per cycle/1  "Freq"
  Correction subsystem/1(Out) -> Sum5/2
  Step/1 -> Switch/2

== system Basics/SM_WT1/Wind Type IV Detailed v2.1 - 9/Control/Measurement and Transformation/Discrete 3-phase PLL-Driven Positive-Sequence Active & Reactive Power/Discrete 3-phase PLL-Driven Positive-Sequence Fundamental Value2/Discrete Variable Frequency Mean value2 ==
  note: Variable frequency - Discrete Mean Value
  note: Pierre Giroux, Gilbert Sybille, Richard Gagnon
      | Power System Simulation Laboratory
      | IREQ, Hydro-Quebc
  Freq : Inport  PortDimensions=1
  In : Inport  Port=2  PortDimensions=1
  Correction subsystem : Subsystem
  Discrete Variable Transport Delay : Subsystem  mask(Discrete variable transport delay){MaxDelay=MaxDelay, InitialValue=0, Ts=Ts}
      mask prompts: MaxDelay "Maximum delay (s):"; InitialValue "Initial input:"; Ts "Sample time:"
      mask help:
      | Apply a delay to the first input (In) signal.
      | The second input (D) specifies the delay time.
  Gain : Gain  Gain=Ts  SaturateOnIntegerOverflow=on  OutDataTypeStr=Inherit: Same as input  ParamDataTypeStr=Inherit: Same as input
  Integ4 : DiscreteIntegrator  IntegratorMethod=Integration: Trapezoidal  SampleTime=Ts  ICPrevOutput=DiscIntNeverNeededParam  ICPrevScaledInput=DiscIntNeverNeededParam
  Number of samples per cycle : Fcn  Expr=1/u[1]/Ts
  Product : Product  SaturateOnIntegerOverflow=on  InputSameDT=on  OutDataTypeStr=Inherit: Same as first input
  Rounding Function : Rounding  Operator=ceil
  Step : Step  Time=1/Finit  SampleTime=Ts
  Sum5 : Sum  SaturateOnIntegerOverflow=on  InputSameDT=on  OutDataTypeStr=Inherit: Same as first input
  Sum7 : Sum  Inputs=-+  SaturateOnIntegerOverflow=on  InputSameDT=on  OutDataTypeStr=Inherit: Same as first input
  Switch : Switch  Threshold=0.5  InputSameDT=on
  To avoid division by zero : Saturate  UpperLimit=1e6  LowerLimit=1e-6
  Unit Delay : UnitDelay  InitialCondition=Vinit  SampleTime=Ts  HasFrameUpgradeWarning=on
  Mean : Outport  VectorParamsAs1DForOutWhenUnconnected=on
  wires:
  Step/1 -> Switch/2
  Correction subsystem/1(Out) -> Sum5/2
  To avoid division by zero/1 -> Number of samples per cycle/1  "Freq"
  Switch/1 -> Unit Delay/1, Mean/1
  Unit Delay/1 -> Switch/3
  Sum5/1 -> Switch/1
  Number of samples per cycle/1 -> Correction subsystem/1(N), Rounding Function/1
  Rounding Function/1 -> Correction subsystem/2(F), Gain/1
  Gain/1 -> Discrete Variable Transport Delay/2(D)  "Delay"
  Freq/1 -> To avoid division by zero/1, Product/2  "Freq"
  Integ4/1 -> Sum7/2, Discrete Variable Transport Delay/1(In)
  Sum7/1 -> Product/1
  Discrete Variable Transport Delay/1(Out) -> Sum7/1
  Product/1 -> Sum5/1  "Mean value"
  In/1 -> Correction subsystem/3(In), Integ4/1  "In"

== system Basics/SM_WT1/Wind Type IV Detailed v2.1 - 1/Control/Measurement and Transformation/Discrete 3-phase PLL-Driven Positive-Sequence Active & Reactive Power/Discrete 3-phase PLL-Driven Positive-Sequence Fundamental Value/Discrete Variable Frequency Mean value1/Correction subsystem ==
  N : Inport
  F : Inport  Port=2
  In : Inport  Port=3
  Gain1 : Gain  Gain=0.5  SaturateOnIntegerOverflow=on  OutDataTypeStr=Inherit: Same as input  ParamDataTypeStr=Inherit: Same as input
  Product2 : Product  Inputs=*/  SaturateOnIntegerOverflow=on  InputSameDT=on  OutDataTypeStr=Inherit: Same as first input
  Product4 : Product  Inputs=**  SaturateOnIntegerOverflow=on  InputSameDT=on  OutDataTypeStr=Inherit: Same as first input
  Product5 : Product  Inputs=**  SaturateOnIntegerOverflow=on  InputSameDT=on  OutDataTypeStr=Inherit: Same as first input
  Sum1 : Sum  Inputs=+-  SaturateOnIntegerOverflow=on  InputSameDT=on  OutDataTypeStr=Inherit: Same as first input
  Sum4 : Sum  SaturateOnIntegerOverflow=on  InputSameDT=on  OutDataTypeStr=Inherit: Same as first input
  Sum5 : Sum  Inputs=+-  SaturateOnIntegerOverflow=on  InputSameDT=on  OutDataTypeStr=Inherit: Same as first input
  Unit Delay : UnitDelay  SampleTime=Ts  HasFrameUpgradeWarning=on
  Out : Outport  VectorParamsAs1DForOutWhenUnconnected=on
  wires:
  Product4/1 -> Out/1
  Sum4/1 -> Product4/2
  Gain1/1 -> Sum4/1
  Product5/1 -> Gain1/1
  Sum1/1 -> Product5/2
  In/1 -> Sum4/2, Unit Delay/1, Sum1/1
  Product2/1 -> Product4/1
  Sum5/1 -> Product5/1, Product2/1
  F/1 -> Sum5/2
  N/1 -> Product2/2, Sum5/1
  Unit Delay/1 -> Sum1/2

== system Basics/SM_WT1/Wind Type IV Detailed v2.1 - 1/Control/Measurement and Transformation/Discrete 3-phase PLL-Driven Positive-Sequence Active & Reactive Power/Discrete 3-phase PLL-Driven Positive-Sequence Fundamental Value/Discrete Variable Frequency Mean value1/Discrete Variable Transport Delay ==
  In : Inport
  D : Inport  Port=2
  "S-Function " : S-Function  FunctionName=discreteVariableTransportDelay  Parameters=MaxDelay,Ts,InitialValue  SFunctionDeploymentMode=off  EnableBusSupport=off
  Out : Outport  VectorParamsAs1DForOutWhenUnconnected=on
  wires:
  D/1 -> "S-Function "/2
  In/1 -> "S-Function "/1
  "S-Function "/1 -> Out/1

== system Basics/SM_WT1/Wind Type IV Detailed v2.1 - 1/Control/Measurement and Transformation/Discrete 3-phase PLL-Driven Positive-Sequence Active & Reactive Power/Discrete 3-phase PLL-Driven Positive-Sequence Fundamental Value/Discrete Variable Frequency Mean value2/Correction subsystem ==
  N : Inport
  F : Inport  Port=2
  In : Inport  Port=3
  Gain1 : Gain  Gain=0.5  SaturateOnIntegerOverflow=on  OutDataTypeStr=Inherit: Same as input  ParamDataTypeStr=Inherit: Same as input
  Product2 : Product  Inputs=*/  SaturateOnIntegerOverflow=on  InputSameDT=on  OutDataTypeStr=Inherit: Same as first input
  Product4 : Product  Inputs=**  SaturateOnIntegerOverflow=on  InputSameDT=on  OutDataTypeStr=Inherit: Same as first input
  Product5 : Product  Inputs=**  SaturateOnIntegerOverflow=on  InputSameDT=on  OutDataTypeStr=Inherit: Same as first input
  Sum1 : Sum  Inputs=+-  SaturateOnIntegerOverflow=on  InputSameDT=on  OutDataTypeStr=Inherit: Same as first input
  Sum4 : Sum  SaturateOnIntegerOverflow=on  InputSameDT=on  OutDataTypeStr=Inherit: Same as first input
  Sum5 : Sum  Inputs=+-  SaturateOnIntegerOverflow=on  InputSameDT=on  OutDataTypeStr=Inherit: Same as first input
  Unit Delay : UnitDelay  SampleTime=Ts  HasFrameUpgradeWarning=on
  Out : Outport  VectorParamsAs1DForOutWhenUnconnected=on
  wires:
  Unit Delay/1 -> Sum1/2
  N/1 -> Sum5/1, Product2/2
  F/1 -> Sum5/2
  Sum5/1 -> Product2/1, Product5/1
  Product2/1 -> Product4/1
  In/1 -> Sum1/1, Unit Delay/1, Sum4/2
  Sum1/1 -> Product5/2
  Product5/1 -> Gain1/1
  Gain1/1 -> Sum4/1
  Sum4/1 -> Product4/2
  Product4/1 -> Out/1

== system Basics/SM_WT1/Wind Type IV Detailed v2.1 - 1/Control/Measurement and Transformation/Discrete 3-phase PLL-Driven Positive-Sequence Active & Reactive Power/Discrete 3-phase PLL-Driven Positive-Sequence Fundamental Value/Discrete Variable Frequency Mean value2/Discrete Variable Transport Delay ==
  In : Inport
  D : Inport  Port=2
  "S-Function " : S-Function  FunctionName=discreteVariableTransportDelay  Parameters=MaxDelay,Ts,InitialValue  SFunctionDeploymentMode=off  EnableBusSupport=off
  Out : Outport  VectorParamsAs1DForOutWhenUnconnected=on
  wires:
  "S-Function "/1 -> Out/1
  In/1 -> "S-Function "/1
  D/1 -> "S-Function "/2

== system Basics/SM_WT1/Wind Type IV Detailed v2.1 - 1/Control/Measurement and Transformation/Discrete 3-phase PLL-Driven Positive-Sequence Active & Reactive Power/Discrete 3-phase PLL-Driven Positive-Sequence Fundamental Value2/Discrete Variable Frequency Mean value1/Correction subsystem ==
  N : Inport
  F : Inport  Port=2
  In : Inport  Port=3
  Gain1 : Gain  Gain=0.5  SaturateOnIntegerOverflow=on  OutDataTypeStr=Inherit: Same as input  ParamDataTypeStr=Inherit: Same as input
  Product2 : Product  Inputs=*/  SaturateOnIntegerOverflow=on  InputSameDT=on  OutDataTypeStr=Inherit: Same as first input
  Product4 : Product  Inputs=**  SaturateOnIntegerOverflow=on  InputSameDT=on  OutDataTypeStr=Inherit: Same as first input
  Product5 : Product  Inputs=**  SaturateOnIntegerOverflow=on  InputSameDT=on  OutDataTypeStr=Inherit: Same as first input
  Sum1 : Sum  Inputs=+-  SaturateOnIntegerOverflow=on  InputSameDT=on  OutDataTypeStr=Inherit: Same as first input
  Sum4 : Sum  SaturateOnIntegerOverflow=on  InputSameDT=on  OutDataTypeStr=Inherit: Same as first input
  Sum5 : Sum  Inputs=+-  SaturateOnIntegerOverflow=on  InputSameDT=on  OutDataTypeStr=Inherit: Same as first input
  Unit Delay : UnitDelay  SampleTime=Ts  HasFrameUpgradeWarning=on
  Out : Outport  VectorParamsAs1DForOutWhenUnconnected=on
  wires:
  Unit Delay/1 -> Sum1/2
  N/1 -> Sum5/1, Product2/2
  F/1 -> Sum5/2
  Sum5/1 -> Product2/1, Product5/1
  Product2/1 -> Product4/1
  In/1 -> Sum1/1, Unit Delay/1, Sum4/2
  Sum1/1 -> Product5/2
  Product5/1 -> Gain1/1
  Gain1/1 -> Sum4/1
  Sum4/1 -> Product4/2
  Product4/1 -> Out/1

== system Basics/SM_WT1/Wind Type IV Detailed v2.1 - 1/Control/Measurement and Transformation/Discrete 3-phase PLL-Driven Positive-Sequence Active & Reactive Power/Discrete 3-phase PLL-Driven Positive-Sequence Fundamental Value2/Discrete Variable Frequency Mean value1/Discrete Variable Transport Delay ==
  In : Inport
  D : Inport  Port=2
  "S-Function " : S-Function  FunctionName=discreteVariableTransportDelay  Parameters=MaxDelay,Ts,InitialValue  SFunctionDeploymentMode=off  EnableBusSupport=off
  Out : Outport  VectorParamsAs1DForOutWhenUnconnected=on
  wires:
  "S-Function "/1 -> Out/1
  In/1 -> "S-Function "/1
  D/1 -> "S-Function "/2

== system Basics/SM_WT1/Wind Type IV Detailed v2.1 - 1/Control/Measurement and Transformation/Discrete 3-phase PLL-Driven Positive-Sequence Active & Reactive Power/Discrete 3-phase PLL-Driven Positive-Sequence Fundamental Value2/Discrete Variable Frequency Mean value2/Correction subsystem ==
  N : Inport
  F : Inport  Port=2
  In : Inport  Port=3
  Gain1 : Gain  Gain=0.5  SaturateOnIntegerOverflow=on  OutDataTypeStr=Inherit: Same as input  ParamDataTypeStr=Inherit: Same as input
  Product2 : Product  Inputs=*/  SaturateOnIntegerOverflow=on  InputSameDT=on  OutDataTypeStr=Inherit: Same as first input
  Product4 : Product  Inputs=**  SaturateOnIntegerOverflow=on  InputSameDT=on  OutDataTypeStr=Inherit: Same as first input
  Product5 : Product  Inputs=**  SaturateOnIntegerOverflow=on  InputSameDT=on  OutDataTypeStr=Inherit: Same as first input
  Sum1 : Sum  Inputs=+-  SaturateOnIntegerOverflow=on  InputSameDT=on  OutDataTypeStr=Inherit: Same as first input
  Sum4 : Sum  SaturateOnIntegerOverflow=on  InputSameDT=on  OutDataTypeStr=Inherit: Same as first input
  Sum5 : Sum  Inputs=+-  SaturateOnIntegerOverflow=on  InputSameDT=on  OutDataTypeStr=Inherit: Same as first input
  Unit Delay : UnitDelay  SampleTime=Ts  HasFrameUpgradeWarning=on
  Out : Outport  VectorParamsAs1DForOutWhenUnconnected=on
  wires:
  Product4/1 -> Out/1
  Sum4/1 -> Product4/2
  Gain1/1 -> Sum4/1
  Product5/1 -> Gain1/1
  Sum1/1 -> Product5/2
  In/1 -> Sum4/2, Unit Delay/1, Sum1/1
  Product2/1 -> Product4/1
  Sum5/1 -> Product5/1, Product2/1
  F/1 -> Sum5/2
  N/1 -> Product2/2, Sum5/1
  Unit Delay/1 -> Sum1/2

== system Basics/SM_WT1/Wind Type IV Detailed v2.1 - 1/Control/Measurement and Transformation/Discrete 3-phase PLL-Driven Positive-Sequence Active & Reactive Power/Discrete 3-phase PLL-Driven Positive-Sequence Fundamental Value2/Discrete Variable Frequency Mean value2/Discrete Variable Transport Delay ==
  In : Inport
  D : Inport  Port=2
  "S-Function " : S-Function  FunctionName=discreteVariableTransportDelay  Parameters=MaxDelay,Ts,InitialValue  SFunctionDeploymentMode=off  EnableBusSupport=off
  Out : Outport  VectorParamsAs1DForOutWhenUnconnected=on
  wires:
  D/1 -> "S-Function "/2
  In/1 -> "S-Function "/1
  "S-Function "/1 -> Out/1

== system Basics/SM_WT1/Wind Type IV Detailed v2.1 - 2/Control/Measurement and Transformation/Discrete 3-phase PLL-Driven Positive-Sequence Active & Reactive Power/Discrete 3-phase PLL-Driven Positive-Sequence Fundamental Value/Discrete Variable Frequency Mean value1/Correction subsystem ==
  N : Inport
  F : Inport  Port=2
  In : Inport  Port=3
  Gain1 : Gain  Gain=0.5  SaturateOnIntegerOverflow=on  OutDataTypeStr=Inherit: Same as input  ParamDataTypeStr=Inherit: Same as input
  Product2 : Product  Inputs=*/  SaturateOnIntegerOverflow=on  InputSameDT=on  OutDataTypeStr=Inherit: Same as first input
  Product4 : Product  Inputs=**  SaturateOnIntegerOverflow=on  InputSameDT=on  OutDataTypeStr=Inherit: Same as first input
  Product5 : Product  Inputs=**  SaturateOnIntegerOverflow=on  InputSameDT=on  OutDataTypeStr=Inherit: Same as first input
  Sum1 : Sum  Inputs=+-  SaturateOnIntegerOverflow=on  InputSameDT=on  OutDataTypeStr=Inherit: Same as first input
  Sum4 : Sum  SaturateOnIntegerOverflow=on  InputSameDT=on  OutDataTypeStr=Inherit: Same as first input
  Sum5 : Sum  Inputs=+-  SaturateOnIntegerOverflow=on  InputSameDT=on  OutDataTypeStr=Inherit: Same as first input
  Unit Delay : UnitDelay  SampleTime=Ts  HasFrameUpgradeWarning=on
  Out : Outport  VectorParamsAs1DForOutWhenUnconnected=on
  wires:
  Unit Delay/1 -> Sum1/2
  N/1 -> Sum5/1, Product2/2
  F/1 -> Sum5/2
  Sum5/1 -> Product2/1, Product5/1
  Product2/1 -> Product4/1
  In/1 -> Sum1/1, Unit Delay/1, Sum4/2
  Sum1/1 -> Product5/2
  Product5/1 -> Gain1/1
  Gain1/1 -> Sum4/1
  Sum4/1 -> Product4/2
  Product4/1 -> Out/1

== system Basics/SM_WT1/Wind Type IV Detailed v2.1 - 2/Control/Measurement and Transformation/Discrete 3-phase PLL-Driven Positive-Sequence Active & Reactive Power/Discrete 3-phase PLL-Driven Positive-Sequence Fundamental Value/Discrete Variable Frequency Mean value1/Discrete Variable Transport Delay ==
  In : Inport
  D : Inport  Port=2
  "S-Function " : S-Function  FunctionName=discreteVariableTransportDelay  Parameters=MaxDelay,Ts,InitialValue  SFunctionDeploymentMode=off  EnableBusSupport=off
  Out : Outport  VectorParamsAs1DForOutWhenUnconnected=on
  wires:
  "S-Function "/1 -> Out/1
  In/1 -> "S-Function "/1
  D/1 -> "S-Function "/2

== system Basics/SM_WT1/Wind Type IV Detailed v2.1 - 2/Control/Measurement and Transformation/Discrete 3-phase PLL-Driven Positive-Sequence Active & Reactive Power/Discrete 3-phase PLL-Driven Positive-Sequence Fundamental Value/Discrete Variable Frequency Mean value2/Correction subsystem ==
  N : Inport
  F : Inport  Port=2
  In : Inport  Port=3
  Gain1 : Gain  Gain=0.5  SaturateOnIntegerOverflow=on  OutDataTypeStr=Inherit: Same as input  ParamDataTypeStr=Inherit: Same as input
  Product2 : Product  Inputs=*/  SaturateOnIntegerOverflow=on  InputSameDT=on  OutDataTypeStr=Inherit: Same as first input
  Product4 : Product  Inputs=**  SaturateOnIntegerOverflow=on  InputSameDT=on  OutDataTypeStr=Inherit: Same as first input
  Product5 : Product  Inputs=**  SaturateOnIntegerOverflow=on  InputSameDT=on  OutDataTypeStr=Inherit: Same as first input
  Sum1 : Sum  Inputs=+-  SaturateOnIntegerOverflow=on  InputSameDT=on  OutDataTypeStr=Inherit: Same as first input
  Sum4 : Sum  SaturateOnIntegerOverflow=on  InputSameDT=on  OutDataTypeStr=Inherit: Same as first input
  Sum5 : Sum  Inputs=+-  SaturateOnIntegerOverflow=on  InputSameDT=on  OutDataTypeStr=Inherit: Same as first input
  Unit Delay : UnitDelay  SampleTime=Ts  HasFrameUpgradeWarning=on
  Out : Outport  VectorParamsAs1DForOutWhenUnconnected=on
  wires:
  Product4/1 -> Out/1
  Sum4/1 -> Product4/2
  Gain1/1 -> Sum4/1
  Product5/1 -> Gain1/1
  Sum1/1 -> Product5/2
  In/1 -> Sum4/2, Unit Delay/1, Sum1/1
  Product2/1 -> Product4/1
  Sum5/1 -> Product5/1, Product2/1
  F/1 -> Sum5/2
  N/1 -> Product2/2, Sum5/1
  Unit Delay/1 -> Sum1/2

== system Basics/SM_WT1/Wind Type IV Detailed v2.1 - 2/Control/Measurement and Transformation/Discrete 3-phase PLL-Driven Positive-Sequence Active & Reactive Power/Discrete 3-phase PLL-Driven Positive-Sequence Fundamental Value/Discrete Variable Frequency Mean value2/Discrete Variable Transport Delay ==
  In : Inport
  D : Inport  Port=2
  "S-Function " : S-Function  FunctionName=discreteVariableTransportDelay  Parameters=MaxDelay,Ts,InitialValue  SFunctionDeploymentMode=off  EnableBusSupport=off
  Out : Outport  VectorParamsAs1DForOutWhenUnconnected=on
  wires:
  D/1 -> "S-Function "/2
  In/1 -> "S-Function "/1
  "S-Function "/1 -> Out/1

== system Basics/SM_WT1/Wind Type IV Detailed v2.1 - 2/Control/Measurement and Transformation/Discrete 3-phase PLL-Driven Positive-Sequence Active & Reactive Power/Discrete 3-phase PLL-Driven Positive-Sequence Fundamental Value2/Discrete Variable Frequency Mean value1/Correction subsystem ==
  N : Inport
  F : Inport  Port=2
  In : Inport  Port=3
  Gain1 : Gain  Gain=0.5  SaturateOnIntegerOverflow=on  OutDataTypeStr=Inherit: Same as input  ParamDataTypeStr=Inherit: Same as input
  Product2 : Product  Inputs=*/  SaturateOnIntegerOverflow=on  InputSameDT=on  OutDataTypeStr=Inherit: Same as first input
  Product4 : Product  Inputs=**  SaturateOnIntegerOverflow=on  InputSameDT=on  OutDataTypeStr=Inherit: Same as first input
  Product5 : Product  Inputs=**  SaturateOnIntegerOverflow=on  InputSameDT=on  OutDataTypeStr=Inherit: Same as first input
  Sum1 : Sum  Inputs=+-  SaturateOnIntegerOverflow=on  InputSameDT=on  OutDataTypeStr=Inherit: Same as first input
  Sum4 : Sum  SaturateOnIntegerOverflow=on  InputSameDT=on  OutDataTypeStr=Inherit: Same as first input
  Sum5 : Sum  Inputs=+-  SaturateOnIntegerOverflow=on  InputSameDT=on  OutDataTypeStr=Inherit: Same as first input
  Unit Delay : UnitDelay  SampleTime=Ts  HasFrameUpgradeWarning=on
  Out : Outport  VectorParamsAs1DForOutWhenUnconnected=on
  wires:
  Product4/1 -> Out/1
  Sum4/1 -> Product4/2
  Gain1/1 -> Sum4/1
  Product5/1 -> Gain1/1
  Sum1/1 -> Product5/2
  In/1 -> Sum4/2, Unit Delay/1, Sum1/1
  Product2/1 -> Product4/1
  Sum5/1 -> Product5/1, Product2/1
  F/1 -> Sum5/2
  N/1 -> Product2/2, Sum5/1
  Unit Delay/1 -> Sum1/2

== system Basics/SM_WT1/Wind Type IV Detailed v2.1 - 2/Control/Measurement and Transformation/Discrete 3-phase PLL-Driven Positive-Sequence Active & Reactive Power/Discrete 3-phase PLL-Driven Positive-Sequence Fundamental Value2/Discrete Variable Frequency Mean value1/Discrete Variable Transport Delay ==
  In : Inport
  D : Inport  Port=2
  "S-Function " : S-Function  FunctionName=discreteVariableTransportDelay  Parameters=MaxDelay,Ts,InitialValue  SFunctionDeploymentMode=off  EnableBusSupport=off
  Out : Outport  VectorParamsAs1DForOutWhenUnconnected=on
  wires:
  D/1 -> "S-Function "/2
  In/1 -> "S-Function "/1
  "S-Function "/1 -> Out/1
